simulink subsystem "SpaceRobot_Dyn"  (R2022a)
settings: Solver=VariableStepAuto  StartTime=0.0  StopTime=10.0  RelTol=1e-3
model mask{spaceRobot=sc}
settings Model: Creator=charl  LastModifiedBy=charl

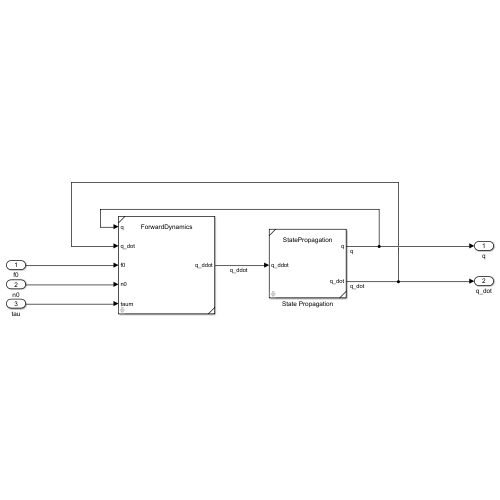
[thumbnail: Simulink's stored preview of the top-level diagram]
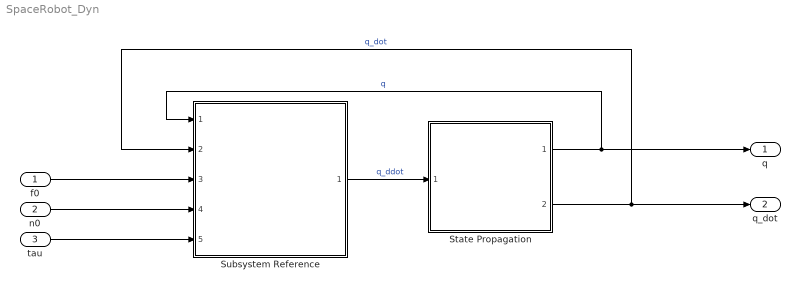
== system SpaceRobot_Dyn ==
  f0 : Inport
  n0 : Inport  Port=2
  tau : Inport  Port=3
  State Propagation : Subsystem  ReferencedSubsystem=StatePropagation  spaceRobot=sc
  Subsystem Reference : Subsystem  ReferencedSubsystem=ForwardDynamics  spaceRobot=spaceRobot  SimulateUsing=Interpreted execution
  q : Outport
  q_dot : Outport  Port=2
  wires:
  f0/1 -> Subsystem Reference/3
  State Propagation/1 -> q/1, Subsystem Reference/1  "q"
  State Propagation/2 -> q_dot/1, Subsystem Reference/2  "q_dot"
  n0/1 -> Subsystem Reference/4
  Subsystem Reference/1 -> State Propagation/1  "q_ddot"
  tau/1 -> Subsystem Reference/5
